simulink model "LQR_pade_observer_discrete"  (R2023b)
settings: Solver=VariableStepAuto  StartTime=0.0  StopTime=40000  FixedStep=Ts  RelTol=1e-3
undefined symbols (not defined in the file): A, B, C, disturbance, K_tilde, kr, L, num_int, sys_discrete, Ts
libraries: cstblocks x2, eeStairGenerator x1
settings Model: SimulationMode=rapid-accelerator  Creator=giova  LastModifiedBy=giova

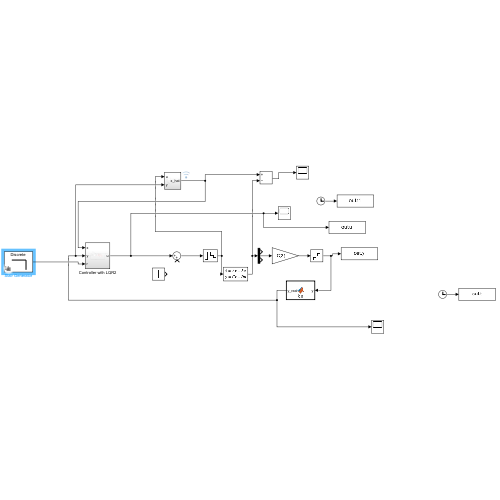
[thumbnail: Simulink's stored preview of the top-level diagram]
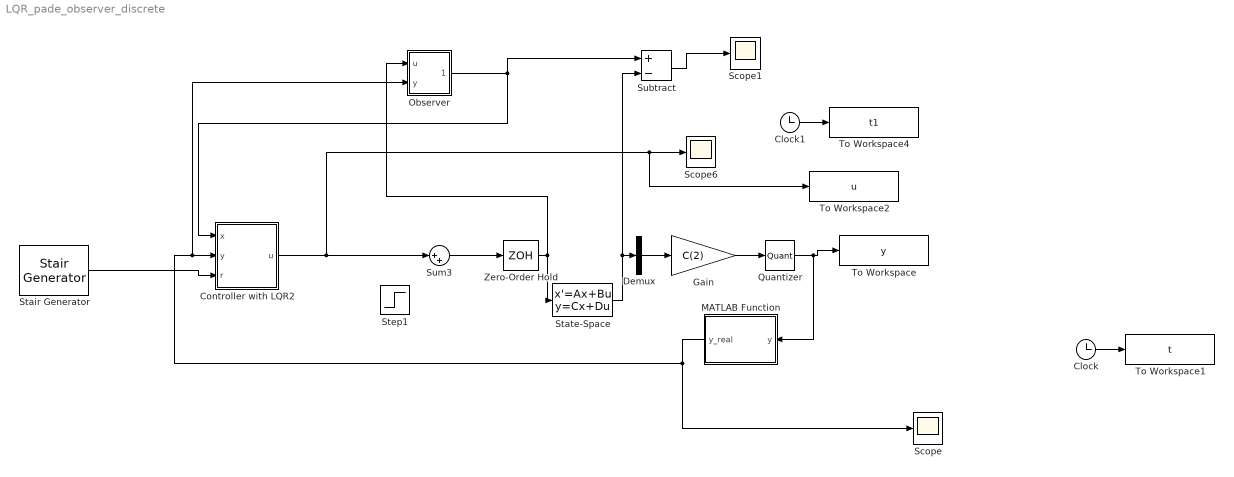
== system LQR_pade_observer_discrete ==
  Clock : Clock
  Clock1 : Clock
  Controller with LQR2 : Subsystem
  Demux : Demux  Outputs=3
  Gain : Gain  Gain=C(2)
  MATLAB Function : MATLAB Function  TreatAsAtomicUnit=on
  Observer : Subsystem
  Quantizer : Quantizer  QuantizationInterval=Ts
  Scope : Scope
  Scope1 : Scope
  Scope6 : Scope
  Stair Generator : eeStairGenerator/Stair Generator  LabelModeActiveChoice=Discrete  TimeInput=[0 20]  AmplitudeInput=[10 pi]  SampleTime=Ts  RepeatPattern=off  OutDataTypeStr=double
      settings: LibrarySourceBlock=ee_sl_lib/General Control/Stair Generator
  State-Space : StateSpace  A=A  B=B  C=eye(3)  D=[0;0;0]  InitialCondition=0
  Step1 : Step  Time=2  After=disturbance  SampleTime=0
  Subtract : Sum  Inputs=+-
  Sum3 : Sum  Inputs=|++
  To Workspace : ToWorkspace  VariableName=y  SampleTime=-1
  To Workspace1 : ToWorkspace  VariableName=t  SampleTime=-1
  To Workspace2 : ToWorkspace  VariableName=u  SampleTime=-1
  To Workspace4 : ToWorkspace  VariableName=t1  SampleTime=-1
  Zero-Order Hold : ZeroOrderHold  SampleTime=Ts
  wires:
  Sum3/1 -> Zero-Order Hold/1
  Controller with LQR2/1(u) -> To Workspace2/1, Scope6/1, Sum3/1
  Clock/1 -> To Workspace1/1
  Clock1/1 -> To Workspace4/1
  Observer/1(x_hat) -> Controller with LQR2/1(x), Subtract/1
  Demux/2 -> Gain/1
  Subtract/1 -> Scope1/1
  Gain/1 -> Quantizer/1
  Quantizer/1 -> MATLAB Function/1(y), To Workspace/1
  State-Space/1 -> Subtract/2, Demux/1
  Zero-Order Hold/1 -> Observer/1(u), State-Space/1
  Stair Generator/1 -> Controller with LQR2/3(r)
  MATLAB Function/1(y_real) -> Observer/2(y), Controller with LQR2/2(y), Scope/1

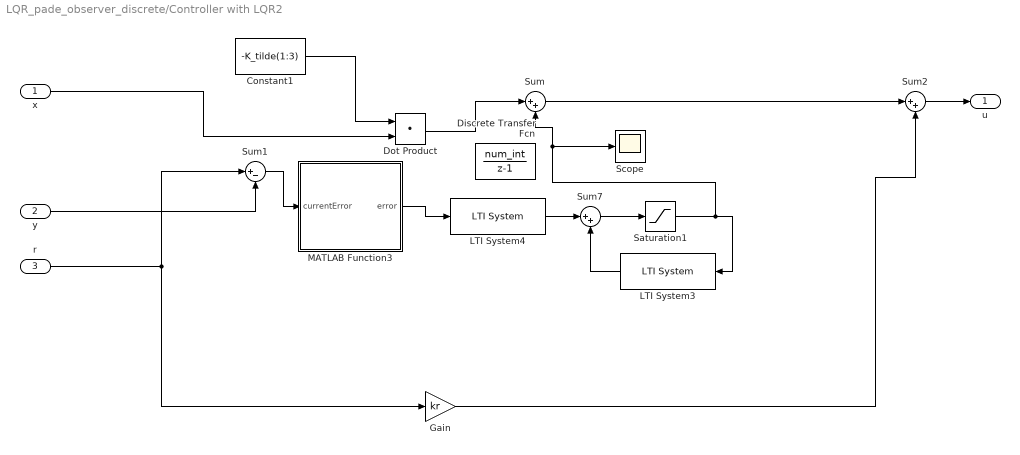
== system LQR_pade_observer_discrete/Controller with LQR2 ==
  x : Inport
  y : Inport  Port=2
  r : Inport  Port=3
  Constant1 : Constant  Value=-K_tilde(1:3)
  Discrete Transfer Fcn : DiscreteTransferFcn  Numerator=num_int  Denominator=[1 -1]
  Dot Product : DotProduct  OutDataTypeStr=Inherit: Inherit via internal rule
  Gain : Gain  Gain=kr
  LTI System3 : cstblocks/LTI System  sys=z_antiwindupFunc  IC=[]  PadeOrder=0
  LTI System4 : cstblocks/LTI System  sys=z_Q_Gamma  IC=[]  PadeOrder=0
  MATLAB Function3 : MATLAB Function  TreatAsAtomicUnit=on
  Saturation1 : Saturate  UpperLimit=12  LowerLimit=-12
  Scope : Scope
  Sum : Sum  Inputs=|++
  Sum1 : Sum  Inputs=|+-
  Sum2 : Sum  Inputs=|++
  Sum7 : Sum  Inputs=|++
  u : Outport
  wires:
  Dot Product/1 -> Sum/1
  y/1 -> Sum1/2
  x/1 -> Dot Product/2
  Sum2/1 -> u/1
  Constant1/1 -> Dot Product/1
  Gain/1 -> Sum2/2
  Sum/1 -> Sum2/1
  r/1 -> Gain/1, Sum1/1
  Sum1/1 -> MATLAB Function3/1(currentError)
  LTI System3/1 -> Sum7/2
  LTI System4/1 -> Sum7/1
  Saturation1/1 -> Scope/1, Sum/2, LTI System3/1
  Sum7/1 -> Saturation1/1
  MATLAB Function3/1(error) -> LTI System4/1

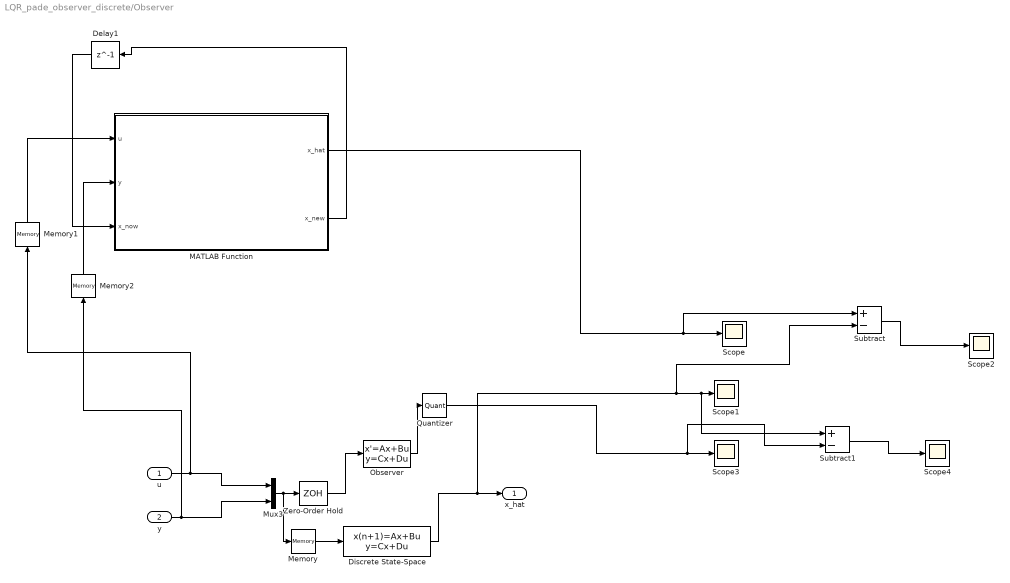
== system LQR_pade_observer_discrete/Observer ==
  u : Inport
  y : Inport  Port=2
  Delay1 : Delay  DelayLength=1  InitialCondition=[0.0 ;0.0 ;0.0]  SampleTime=Ts
  Discrete State-Space : DiscreteStateSpace  A=sys_discrete.A  B=sys_discrete.B  C=sys_discrete.C  D=sys_discrete.D  SampleTime=Ts
  MATLAB Function : MATLAB Function  TreatAsAtomicUnit=on
  Memory : Memory
  Memory1 : Memory
  Memory2 : Memory
  Mux3 : Mux  Inputs=2
  Observer : StateSpace  A=A-L*C  B=[B L]  C=eye(3)  D=[0 0; 0 0; 0 0]  InitialCondition=[0 0 0]  ParameterTunability=Unconstrained
  Quantizer : Quantizer  QuantizationInterval=Ts
  Scope{,1..4} (5 alike) : Scope
  Subtract : Sum  Inputs=+-
  Subtract1 : Sum  Inputs=+-
  Zero-Order Hold : ZeroOrderHold  SampleTime=-1
  x_hat : Outport
  wires:
  y/1 -> Mux3/2, Memory2/1
  u/1 -> Mux3/1, Memory1/1
  Mux3/1 -> Memory/1, Zero-Order Hold/1
  Zero-Order Hold/1 -> Observer/1
  Discrete State-Space/1 -> Subtract/2, Subtract1/1, Scope1/1, x_hat/1
  Observer/1 -> Quantizer/1
  Memory/1 -> Discrete State-Space/1
  Delay1/1 -> MATLAB Function/3(x_now)
  MATLAB Function/2(x_new) -> Delay1/1
  MATLAB Function/1(x_hat) -> Subtract/1, Scope/1
  Subtract/1 -> Scope2/1
  Quantizer/1 -> Subtract1/2, Scope3/1
  Subtract1/1 -> Scope4/1
  Memory2/1 -> MATLAB Function/2(y)
  Memory1/1 -> MATLAB Function/1(u)

== matlab function LQR_pade_observer_discrete/MATLAB Function ==
  data: y input; y_real output
function y_real = fcn(y)
    y_real = sign(y)*mod(abs(y),2*pi);
end

== matlab function LQR_pade_observer_discrete/Controller with LQR2/MATLAB Function3 ==
  data: currentError input; error output
function error = getErrorPos(currentError)

error=currentError;
if (currentError>pi)
    error = currentError-2*pi;
end

if(currentError<-pi)
    error = currentError + 2*pi;
end

end

== matlab function LQR_pade_observer_discrete/Observer/MATLAB Function ==
  data: u input; x_hat output; y input; x_new output; x_now input
function [x_hat,x_new]= fcn(u, y, x_now)
A = [0.9323301716064688  -11.678660637721487    0.039014496138124237;
    0.0027413091396064947    0.1183557159613379    5.5348095481874759e-5;
   -0.0068954979109303533   -2.8131155992845822    0.8383381318909956];

B = [-0.0040505355062536866    2.0794225090756346;
   -5.7463109393787418e-6    0.15697955665449895;
    0.036784001382597235    0.50088414067706177];
    
C = [0.96616508580323435  -5.8393303188607444    0.019507248069062118;
    0.0013706545698032474    0.559177857980669    2.767404774093738e-5;
   -0.0034477489554651771  -1.4065577996422911    0.91916906594549774];

D = [-0.0020252677531268433    1.0397112545378173;
   -2.8731554696893709e-6   0.078489778327249474;
    0.018392000691298618   0.25044207033853089];

x1 = x_now(1);
x2 = x_now(2);
x3 = x_now(3);

x1_stimato = C(1) * x1 + C(4) * x2 + C(7) * x3 + D(1) * u + D(4) * y;
x2_stimato = C(2) * x1 + C(5) * x2 + C(8) * x3 + D(2) * u + D(5) * y;
x3_stimato = C(3) * x1 + C(6) * x2 + C(9) * x3 + D(3) * u + D(6) * y;

x1_new = A(1) * x1 + A(4) * x2 + A(7) * x3 + B(1) * u + B(4) * y;
x2_new = A(2) * x1 + A(5) * x2 + A(8) * x3 + B(2) * u + B(5) * y;
x3_new = A(3) * x1 + A(6) * x2 + A(9) * x3 + B(3) * u + B(6) * y;


x_new = [x1_new ;x2_new ;x3_new];
x_hat = [x1_stimato ;x2_stimato ;x3_stimato];
